simulink library "halout"  (R2021b)
settings: Solver=VariableStepAuto  StartTime=0.0  StopTime=10.0  RelTol=1e-3
undefined symbols (not defined in the file): C_TASK_5MS_S, FALSE, KHAL_CAN1FD1APS3E2E_flg, KHAL_CAN1FD1APS3TxReq_flg, KHAL_CAN1FD1VCU2E2E_flg, KHAL_CAN1FD1VCU2TxReq_flg, KHAL_CAN1FD1VCU3E2E_flg, KHAL_CAN1FD1VCU3TxReq_flg, KHAL_CAN1TxReq_flg, KHAL_CAN1VMCFCM1E2E_flg, KHAL_CAN1VMCFCM1TxReq_flg, KHAL_CAN2TxReq_flg, KHAL_CAN3FD3VCU1toNIDECTxReq_flg, KHAL_CAN3FD3VCU1TxReq_flg, KHAL_CAN3FD3VCU2E2E_flg, KHAL_CAN3FD3VCU2toNIDECE2E_flg, KHAL_CAN3FD3VCU2toNIDECTxReq_flg, KHAL_CAN3FD3VCU2TxReq_flg, KHAL_CAN3TxReq_flg, KHAL_CAN4FD4CE1000E2E_flg, KHAL_CAN4FD4CE1000TxReq_flg, KHAL_CAN4TxReq_flg, KHAL_CAN5TxReq_flg, KHAL_CAN6FD6APS3E2E_flg, KHAL_CAN6FD6APS3TxReq_flg, KHAL_CAN6FD6VCU2E2E_flg, KHAL_CAN6FD6VCU2TxReq_flg, KHAL_CAN6TxReq_flg, ONE_INT, TRUE, ZERO_INT
libraries: FVT_lib x551, simulink x244
(part 17 of 26)

== system halout/HAL_OUT/CAN2/FD2_C20_0_0x210/PASDRCR ==
  PASDRCR : Inport
  Data Type Conversion : DataTypeConversion  OutDataTypeStr=uint8  RndMeth=Round
  CAN2_PAS_D_RCR : Outport
  wires:
  Data Type Conversion/1 -> CAN2_PAS_D_RCR/1
  PASDRCR/1 -> Data Type Conversion/1

== system halout/HAL_OUT/CAN2/FD2_C20_0_0x210/PASDRML ==
  PASDRML : Inport
  Data Type Conversion : DataTypeConversion  OutDataTypeStr=uint8  RndMeth=Round
  CAN2_PAS_D_RML : Outport
  wires:
  Data Type Conversion/1 -> CAN2_PAS_D_RML/1
  PASDRML/1 -> Data Type Conversion/1

== system halout/HAL_OUT/CAN2/FD2_C20_0_0x210/PASDRMR ==
  PASDRMR : Inport
  Data Type Conversion : DataTypeConversion  OutDataTypeStr=uint8  RndMeth=Round
  CAN2_PAS_D_RMR : Outport
  wires:
  Data Type Conversion/1 -> CAN2_PAS_D_RMR/1
  PASDRMR/1 -> Data Type Conversion/1

== system halout/HAL_OUT/CAN2/FD2_C20_0_0x210/PASSNSRLayout ==
  PASSNSRLayout : Inport
  Data Type Conversion : DataTypeConversion  OutDataTypeStr=uint8  RndMeth=Round
  CAN2_PAS_SNSR_Layout : Outport
  wires:
  Data Type Conversion/1 -> CAN2_PAS_SNSR_Layout/1
  PASSNSRLayout/1 -> Data Type Conversion/1

== system halout/HAL_OUT/CAN2/FD2_C20_0_0x210/USSStaFCL ==
  USSStaFCL : Inport
  Data Type Conversion : DataTypeConversion  OutDataTypeStr=uint8  RndMeth=Round
  CAN2_USS_Sta_FCL : Outport
  wires:
  Data Type Conversion/1 -> CAN2_USS_Sta_FCL/1
  USSStaFCL/1 -> Data Type Conversion/1

== system halout/HAL_OUT/CAN2/FD2_C20_0_0x210/USSStaFCR ==
  USSStaFCR : Inport
  Data Type Conversion : DataTypeConversion  OutDataTypeStr=uint8  RndMeth=Round
  CAN2_USS_Sta_FCR : Outport
  wires:
  Data Type Conversion/1 -> CAN2_USS_Sta_FCR/1
  USSStaFCR/1 -> Data Type Conversion/1

== system halout/HAL_OUT/CAN2/FD2_C20_0_0x210/USSStaFLL ==
  USSStaFLL : Inport
  Data Type Conversion : DataTypeConversion  OutDataTypeStr=uint8  RndMeth=Round
  CAN2_USS_Sta_FLL : Outport
  wires:
  Data Type Conversion/1 -> CAN2_USS_Sta_FLL/1
  USSStaFLL/1 -> Data Type Conversion/1

== system halout/HAL_OUT/CAN2/FD2_C20_0_0x210/USSStaFLR ==
  USSStaFLR : Inport
  Data Type Conversion : DataTypeConversion  OutDataTypeStr=uint8  RndMeth=Round
  CAN2_USS_Sta_FLR : Outport
  wires:
  Data Type Conversion/1 -> CAN2_USS_Sta_FLR/1
  USSStaFLR/1 -> Data Type Conversion/1

== system halout/HAL_OUT/CAN2/FD2_C20_0_0x210/USSStaFML ==
  USSStaFML : Inport
  Data Type Conversion : DataTypeConversion  OutDataTypeStr=uint8  RndMeth=Round
  CAN2_USS_Sta_FML : Outport
  wires:
  Data Type Conversion/1 -> CAN2_USS_Sta_FML/1
  USSStaFML/1 -> Data Type Conversion/1

== system halout/HAL_OUT/CAN2/FD2_C20_0_0x210/USSStaFMR ==
  USSStaFMR : Inport
  Data Type Conversion : DataTypeConversion  OutDataTypeStr=uint8  RndMeth=Round
  CAN2_USS_Sta_FMR : Outport
  wires:
  Data Type Conversion/1 -> CAN2_USS_Sta_FMR/1
  USSStaFMR/1 -> Data Type Conversion/1

== system halout/HAL_OUT/CAN2/FD2_C20_0_0x210/USSStaRCL ==
  USSStaRCL : Inport
  Data Type Conversion : DataTypeConversion  OutDataTypeStr=uint8  RndMeth=Round
  CAN2_USS_Sta_RCL : Outport
  wires:
  Data Type Conversion/1 -> CAN2_USS_Sta_RCL/1
  USSStaRCL/1 -> Data Type Conversion/1

== system halout/HAL_OUT/CAN2/FD2_C20_0_0x210/USSStaRCR ==
  USSStaRCR : Inport
  Data Type Conversion : DataTypeConversion  OutDataTypeStr=uint8  RndMeth=Round
  CAN2_USS_Sta_RCR : Outport
  wires:
  Data Type Conversion/1 -> CAN2_USS_Sta_RCR/1
  USSStaRCR/1 -> Data Type Conversion/1

== system halout/HAL_OUT/CAN2/FD2_C20_0_0x210/USSStaRLL ==
  USSStaRLL : Inport
  Data Type Conversion : DataTypeConversion  OutDataTypeStr=uint8  RndMeth=Round
  CAN2_USS_Sta_RLL : Outport
  wires:
  Data Type Conversion/1 -> CAN2_USS_Sta_RLL/1
  USSStaRLL/1 -> Data Type Conversion/1

== system halout/HAL_OUT/CAN2/FD2_C20_0_0x210/USSStaRLR ==
  USSStaRLR : Inport
  Data Type Conversion : DataTypeConversion  OutDataTypeStr=uint8  RndMeth=Round
  CAN2_USS_Sta_RLR : Outport
  wires:
  Data Type Conversion/1 -> CAN2_USS_Sta_RLR/1
  USSStaRLR/1 -> Data Type Conversion/1

== system halout/HAL_OUT/CAN2/FD2_C20_0_0x210/USSStaRML ==
  USSStaRML : Inport
  Data Type Conversion : DataTypeConversion  OutDataTypeStr=uint8  RndMeth=Round
  CAN2_USS_Sta_RML : Outport
  wires:
  Data Type Conversion/1 -> CAN2_USS_Sta_RML/1
  USSStaRML/1 -> Data Type Conversion/1

== system halout/HAL_OUT/CAN2/FD2_C20_0_0x210/USSStaRMR ==
  USSStaRMR : Inport
  Data Type Conversion : DataTypeConversion  OutDataTypeStr=uint8  RndMeth=Round
  CAN2_USS_Sta_RMR : Outport
  wires:
  Data Type Conversion/1 -> CAN2_USS_Sta_RMR/1
  USSStaRMR/1 -> Data Type Conversion/1

== system halout/HAL_OUT/CAN2/FD2_C20_0_0x210/VMCVCUCCCrlSta ==
  VMCVCUCCCrlSta : Inport
  Data Type Conversion : DataTypeConversion  OutDataTypeStr=uint8  RndMeth=Round
  CAN2_VMC_VCU_CC_Crl_Sta : Outport
  wires:
  Data Type Conversion/1 -> CAN2_VMC_VCU_CC_Crl_Sta/1
  VMCVCUCCCrlSta/1 -> Data Type Conversion/1

== system halout/HAL_OUT/CAN2/FD2_C20_0_0x210/VMCVCUMSACrlSta ==
  VMCVCUMSACrlSta : Inport
  Data Type Conversion : DataTypeConversion  OutDataTypeStr=uint8  RndMeth=Round
  CAN2_VMC_VCU_MSA_Crl_Sta : Outport
  wires:
  Data Type Conversion/1 -> CAN2_VMC_VCU_MSA_Crl_Sta/1
  VMCVCUMSACrlSta/1 -> Data Type Conversion/1

== system halout/HAL_OUT/CAN2/FD2_CE100_0_0x117/APMDoorControlSta ==
  APMDoorControlSta : Inport
  Data Type Conversion : DataTypeConversion  OutDataTypeStr=uint8  RndMeth=Round
  CAN2_APMDoorControlSta : Outport
  wires:
  Data Type Conversion/1 -> CAN2_APMDoorControlSta/1
  APMDoorControlSta/1 -> Data Type Conversion/1

== system halout/HAL_OUT/CAN2/FD2_CE100_0_0x117/ActAPSPosn ==
  ActAPSPosn : Inport
  Data Type Conversion : DataTypeConversion  OutDataTypeStr=uint8  RndMeth=Round
  convert_out : FVT_lib/hal/convert_out  gain=0.394  offset=0
  CAN2_ActAPSPosn : Outport
  wires:
  Data Type Conversion/1 -> CAN2_ActAPSPosn/1
  convert_out/1 -> Data Type Conversion/1
  ActAPSPosn/1 -> convert_out/1

== system halout/HAL_OUT/CAN2/FD2_CE100_0_0x117/AllDoorSW ==
  AllDoorSW : Inport
  Data Type Conversion : DataTypeConversion  OutDataTypeStr=uint8  RndMeth=Round
  CAN2_AllDoorSW : Outport
  wires:
  Data Type Conversion/1 -> CAN2_AllDoorSW/1
  AllDoorSW/1 -> Data Type Conversion/1

== system halout/HAL_OUT/CAN2/FD2_CE100_0_0x117/AntitheftSta ==
  AntitheftSta : Inport
  Data Type Conversion : DataTypeConversion  OutDataTypeStr=uint8  RndMeth=Round
  CAN2_AntitheftSta : Outport
  wires:
  Data Type Conversion/1 -> CAN2_AntitheftSta/1
  AntitheftSta/1 -> Data Type Conversion/1

== system halout/HAL_OUT/CAN2/FD2_CE100_0_0x117/BCMDoorLockSta ==
  BCMDoorLockSta : Inport
  Data Type Conversion : DataTypeConversion  OutDataTypeStr=uint8  RndMeth=Round
  CAN2_BCM_DoorLock_Sta : Outport
  wires:
  Data Type Conversion/1 -> CAN2_BCM_DoorLock_Sta/1
  BCMDoorLockSta/1 -> Data Type Conversion/1

== system halout/HAL_OUT/CAN2/FD2_CE100_0_0x117/BrakeLamp ==
  BrakeLamp : Inport
  Data Type Conversion : DataTypeConversion  OutDataTypeStr=uint8  RndMeth=Round
  CAN2_BrakeLamp : Outport
  wires:
  Data Type Conversion/1 -> CAN2_BrakeLamp/1
  BrakeLamp/1 -> Data Type Conversion/1

== system halout/HAL_OUT/CAN2/FD2_CE100_0_0x117/CCCrlSta ==
  CCCrlSta : Inport
  Data Type Conversion : DataTypeConversion  OutDataTypeStr=uint8  RndMeth=Round
  CAN2_CC_Crl_Sta : Outport
  wires:
  Data Type Conversion/1 -> CAN2_CC_Crl_Sta/1
  CCCrlSta/1 -> Data Type Conversion/1

== system halout/HAL_OUT/CAN2/FD2_CE100_0_0x117/CCMSASpdWar ==
  CCMSASpdWar : Inport
  Data Type Conversion : DataTypeConversion  OutDataTypeStr=uint8  RndMeth=Round
  CAN2_CCMSA_SpdWar : Outport
  wires:
  Data Type Conversion/1 -> CAN2_CCMSA_SpdWar/1
  CCMSASpdWar/1 -> Data Type Conversion/1

== system halout/HAL_OUT/CAN2/FD2_CE100_0_0x117/CCUACLampSts ==
  CCUACLampSts : Inport
  Data Type Conversion : DataTypeConversion  OutDataTypeStr=uint8  RndMeth=Round
  CAN2_CCU_ACLampSts : Outport
  wires:
  Data Type Conversion/1 -> CAN2_CCU_ACLampSts/1
  CCUACLampSts/1 -> Data Type Conversion/1

== system halout/HAL_OUT/CAN2/FD2_CE100_0_0x117/CCUACMaxLampSts ==
  CCUACMaxLampSts : Inport
  Data Type Conversion : DataTypeConversion  OutDataTypeStr=uint8  RndMeth=Round
  CAN2_CCU_ACMaxLampSts : Outport
  wires:
  Data Type Conversion/1 -> CAN2_CCU_ACMaxLampSts/1
  CCUACMaxLampSts/1 -> Data Type Conversion/1

== system halout/HAL_OUT/CAN2/FD2_CE100_0_0x117/CCUAutoLampSts ==
  CCUAutoLampSts : Inport
  Data Type Conversion : DataTypeConversion  OutDataTypeStr=uint8  RndMeth=Round
  CAN2_CCU_AutoLampSts : Outport
  wires:
  Data Type Conversion/1 -> CAN2_CCU_AutoLampSts/1
  CCUAutoLampSts/1 -> Data Type Conversion/1

== system halout/HAL_OUT/CAN2/FD2_CE100_0_0x117/CCUAutoMidLampSts ==
  CCUAutoMidLampSts : Inport
  Data Type Conversion : DataTypeConversion  OutDataTypeStr=uint8  RndMeth=Round
  CAN2_CCU_AutoMidLampSts : Outport
  wires:
  Data Type Conversion/1 -> CAN2_CCU_AutoMidLampSts/1
  CCUAutoMidLampSts/1 -> Data Type Conversion/1

== system halout/HAL_OUT/CAN2/FD2_CE100_0_0x117/CCUDispalyRequest ==
  CCUDispalyRequest : Inport
  Data Type Conversion : DataTypeConversion  OutDataTypeStr=uint8  RndMeth=Round
  CAN2_CCU_Dispaly_Request : Outport
  wires:
  Data Type Conversion/1 -> CAN2_CCU_Dispaly_Request/1
  CCUDispalyRequest/1 -> Data Type Conversion/1

== system halout/HAL_OUT/CAN2/FD2_CE100_0_0x117/CCUEcoSts ==
  CCUEcoSts : Inport
  Data Type Conversion : DataTypeConversion  OutDataTypeStr=uint8  RndMeth=Round
  CAN2_CCU_EcoSts : Outport
  wires:
  Data Type Conversion/1 -> CAN2_CCU_EcoSts/1
  CCUEcoSts/1 -> Data Type Conversion/1

== system halout/HAL_OUT/CAN2/FD2_CE100_0_0x117/CCUFrtOnOffLampSts ==
  CCUFrtOnOffLampSts : Inport
  Data Type Conversion : DataTypeConversion  OutDataTypeStr=uint8  RndMeth=Round
  CAN2_CCU_FrtOnOffLampSts : Outport
  wires:
  Data Type Conversion/1 -> CAN2_CCU_FrtOnOffLampSts/1
  CCUFrtOnOffLampSts/1 -> Data Type Conversion/1

== system halout/HAL_OUT/CAN2/FD2_CE100_0_0x117/CCURrOnOffLampSts ==
  CCURrOnOffLampSts : Inport
  Data Type Conversion : DataTypeConversion  OutDataTypeStr=uint8  RndMeth=Round
  CAN2_CCU_RrOnOffLampSts : Outport
  wires:
  Data Type Conversion/1 -> CAN2_CCU_RrOnOffLampSts/1
  CCURrOnOffLampSts/1 -> Data Type Conversion/1

== system halout/HAL_OUT/CAN2/FD2_CE100_0_0x117/CCUSyncLampSts ==
  CCUSyncLampSts : Inport
  Data Type Conversion : DataTypeConversion  OutDataTypeStr=uint8  RndMeth=Round
  CAN2_CCU_SyncLampSts : Outport
  wires:
  Data Type Conversion/1 -> CAN2_CCU_SyncLampSts/1
  CCUSyncLampSts/1 -> Data Type Conversion/1

== system halout/HAL_OUT/CAN2/FD2_CE100_0_0x117/CoastDwModeStaChk ==
  CoastDwModeStaChk : Inport
  Data Type Conversion : DataTypeConversion  OutDataTypeStr=uint8  RndMeth=Round
  CAN2_CoastDwModeStaChk : Outport
  wires:
  Data Type Conversion/1 -> CAN2_CoastDwModeStaChk/1
  CoastDwModeStaChk/1 -> Data Type Conversion/1

== system halout/HAL_OUT/CAN2/FD2_CE100_0_0x117/CreepSWSta ==
  CreepSWSta : Inport
  Data Type Conversion : DataTypeConversion  OutDataTypeStr=uint8  RndMeth=Round
  CAN2_CreepSW_Sta : Outport
  wires:
  Data Type Conversion/1 -> CAN2_CreepSW_Sta/1
  CreepSWSta/1 -> Data Type Conversion/1

== system halout/HAL_OUT/CAN2/FD2_CE100_0_0x117/DISCButtSta ==
  DISCButtSta : Inport
  Data Type Conversion : DataTypeConversion  OutDataTypeStr=uint8  RndMeth=Round
  CAN2_DISC_ButtSta : Outport
  wires:
  Data Type Conversion/1 -> CAN2_DISC_ButtSta/1
  DISCButtSta/1 -> Data Type Conversion/1

== system halout/HAL_OUT/CAN2/FD2_CE100_0_0x117/DISCSta ==
  DISCSta : Inport
  Data Type Conversion : DataTypeConversion  OutDataTypeStr=uint8  RndMeth=Round
  CAN2_DISC_Sta : Outport
  wires:
  Data Type Conversion/1 -> CAN2_DISC_Sta/1
  DISCSta/1 -> Data Type Conversion/1

== system halout/HAL_OUT/CAN2/FD2_CE100_0_0x117/DemoModeStaChk ==
  DemoModeStaChk : Inport
  Data Type Conversion : DataTypeConversion  OutDataTypeStr=uint8  RndMeth=Round
  CAN2_DemoModeStaChk : Outport
  wires:
  Data Type Conversion/1 -> CAN2_DemoModeStaChk/1
  DemoModeStaChk/1 -> Data Type Conversion/1

== system halout/HAL_OUT/CAN2/FD2_CE100_0_0x117/Dimmer ==
  Dimmer : Inport
  Data Type Conversion : DataTypeConversion  OutDataTypeStr=uint8  RndMeth=Round
  CAN2_Dimmer : Outport
  wires:
  Data Type Conversion/1 -> CAN2_Dimmer/1
  Dimmer/1 -> Data Type Conversion/1

== system halout/HAL_OUT/CAN2/FD2_CE100_0_0x117/DimmerEN ==
  DimmerEN : Inport
  Data Type Conversion : DataTypeConversion  OutDataTypeStr=uint8  RndMeth=Round
  CAN2_DimmerEN : Outport
  wires:
  Data Type Conversion/1 -> CAN2_DimmerEN/1
  DimmerEN/1 -> Data Type Conversion/1

== system halout/HAL_OUT/CAN2/FD2_CE100_0_0x117/DisengagePFail ==
  DisengagePFail : Inport
  Data Type Conversion : DataTypeConversion  OutDataTypeStr=uint8  RndMeth=Round
  CAN2_DisengageP_Fail : Outport
  wires:
  Data Type Conversion/1 -> CAN2_DisengageP_Fail/1
  DisengagePFail/1 -> Data Type Conversion/1

== system halout/HAL_OUT/CAN2/FD2_CE100_0_0x117/DoorLockIND ==
  DoorLockIND : Inport
  Data Type Conversion : DataTypeConversion  OutDataTypeStr=uint8  RndMeth=Round
  CAN2_DoorLockIND : Outport
  wires:
  Data Type Conversion/1 -> CAN2_DoorLockIND/1
  DoorLockIND/1 -> Data Type Conversion/1

== system halout/HAL_OUT/CAN2/FD2_CE100_0_0x117/DrDoorSW ==
  DrDoorSW : Inport
  Data Type Conversion : DataTypeConversion  OutDataTypeStr=uint8  RndMeth=Round
  CAN2_DrDoorSW : Outport
  wires:
  Data Type Conversion/1 -> CAN2_DrDoorSW/1
  DrDoorSW/1 -> Data Type Conversion/1

== system halout/HAL_OUT/CAN2/FD2_CE100_0_0x117/DrSeatSta ==
  DrSeatSta : Inport
  Data Type Conversion : DataTypeConversion  OutDataTypeStr=uint8  RndMeth=Round
  CAN2_Dr_SeatSta : Outport
  wires:
  Data Type Conversion/1 -> CAN2_Dr_SeatSta/1
  DrSeatSta/1 -> Data Type Conversion/1

== system halout/HAL_OUT/CAN2/FD2_CE100_0_0x117/DynoModeStaChk ==
  DynoModeStaChk : Inport
  Data Type Conversion : DataTypeConversion  OutDataTypeStr=uint8  RndMeth=Round
  CAN2_DynoModeStaChk : Outport
  wires:
  Data Type Conversion/1 -> CAN2_DynoModeStaChk/1
  DynoModeStaChk/1 -> Data Type Conversion/1

== system halout/HAL_OUT/CAN2/FD2_CE100_0_0x117/EDriveSysErrAccPedalErr ==
  EDriveSysErrAccPedalErr : Inport
  Data Type Conversion : DataTypeConversion  OutDataTypeStr=uint8  RndMeth=Round
  CAN2_EDriveSysErr_AccPedalErr : Outport
  wires:
  Data Type Conversion/1 -> CAN2_EDriveSysErr_AccPedalErr/1
  EDriveSysErrAccPedalErr/1 -> Data Type Conversion/1

== system halout/HAL_OUT/CAN2/FD2_CE100_0_0x117/EDriveSysErrMCUErr ==
  EDriveSysErrMCUErr : Inport
  Data Type Conversion : DataTypeConversion  OutDataTypeStr=uint8  RndMeth=Round
  CAN2_EDriveSysErr_MCUErr : Outport
  wires:
  Data Type Conversion/1 -> CAN2_EDriveSysErr_MCUErr/1
  EDriveSysErrMCUErr/1 -> Data Type Conversion/1

== system halout/HAL_OUT/CAN2/FD2_CE100_0_0x117/EDriveSysErrShifterErr ==
  EDriveSysErrShifterErr : Inport
  Data Type Conversion : DataTypeConversion  OutDataTypeStr=uint8  RndMeth=Round
  CAN2_EDriveSysErr_ShifterErr : Outport
  wires:
  Data Type Conversion/1 -> CAN2_EDriveSysErr_ShifterErr/1
  EDriveSysErrShifterErr/1 -> Data Type Conversion/1

== system halout/HAL_OUT/CAN2/FD2_CE100_0_0x117/EDriveSysErrVCUErr ==
  EDriveSysErrVCUErr : Inport
  Data Type Conversion : DataTypeConversion  OutDataTypeStr=uint8  RndMeth=Round
  CAN2_EDriveSysErr_VCUErr : Outport
  wires:
  Data Type Conversion/1 -> CAN2_EDriveSysErr_VCUErr/1
  EDriveSysErrVCUErr/1 -> Data Type Conversion/1

== system halout/HAL_OUT/CAN2/FD2_CE100_0_0x117/EVDriveMode ==
  EVDriveMode : Inport
  Data Type Conversion : DataTypeConversion  OutDataTypeStr=uint8  RndMeth=Round
  CAN2_EVDriveMode : Outport
  wires:
  Data Type Conversion/1 -> CAN2_EVDriveMode/1
  EVDriveMode/1 -> Data Type Conversion/1

== system halout/HAL_OUT/CAN2/FD2_CE100_0_0x117/EngAGSCloseSta ==
  EngAGSCloseSta : Inport
  Data Type Conversion : DataTypeConversion  OutDataTypeStr=uint8  RndMeth=Round
  CAN2_Eng_AGSCloseSta : Outport
  wires:
  Data Type Conversion/1 -> CAN2_Eng_AGSCloseSta/1
  EngAGSCloseSta/1 -> Data Type Conversion/1

== system halout/HAL_OUT/CAN2/FD2_CE100_0_0x117/EngActvDmpDisabSta ==
  EngActvDmpDisabSta : Inport
  Data Type Conversion : DataTypeConversion  OutDataTypeStr=uint8  RndMeth=Round
  CAN2_Eng_ActvDmpDisabSta : Outport
  wires:
  Data Type Conversion/1 -> CAN2_Eng_ActvDmpDisabSta/1
  EngActvDmpDisabSta/1 -> Data Type Conversion/1

== system halout/HAL_OUT/CAN2/FD2_CE100_0_0x117/EngCoastDwSta ==
  EngCoastDwSta : Inport
  Data Type Conversion : DataTypeConversion  OutDataTypeStr=uint8  RndMeth=Round
  CAN2_Eng_CoastDwSta : Outport
  wires:
  Data Type Conversion/1 -> CAN2_Eng_CoastDwSta/1
  EngCoastDwSta/1 -> Data Type Conversion/1

== system halout/HAL_OUT/CAN2/FD2_CE100_0_0x117/EngPwrLockSta ==
  EngPwrLockSta : Inport
  Data Type Conversion : DataTypeConversion  OutDataTypeStr=uint8  RndMeth=Round
  CAN2_Eng_PwrLockSta : Outport
  wires:
  Data Type Conversion/1 -> CAN2_Eng_PwrLockSta/1
  EngPwrLockSta/1 -> Data Type Conversion/1

== system halout/HAL_OUT/CAN2/FD2_CE100_0_0x117/EngagePFail ==
  EngagePFail : Inport
  Data Type Conversion : DataTypeConversion  OutDataTypeStr=uint8  RndMeth=Round
  CAN2_EngageP_Fail : Outport
  wires:
  Data Type Conversion/1 -> CAN2_EngageP_Fail/1
  EngagePFail/1 -> Data Type Conversion/1

== system halout/HAL_OUT/CAN2/FD2_CE100_0_0x117/FDABSWarning ==
  FDABSWarning : Inport
  Data Type Conversion : DataTypeConversion  OutDataTypeStr=uint8  RndMeth=Round
  CAN2_FD_ABS_Warning : Outport
  wires:
  Data Type Conversion/1 -> CAN2_FD_ABS_Warning/1
  FDABSWarning/1 -> Data Type Conversion/1

== system halout/HAL_OUT/CAN2/FD2_CE100_0_0x117/FDAGSCmd ==
  FDAGSCmd : Inport
  Data Type Conversion : DataTypeConversion  OutDataTypeStr=uint8  RndMeth=Round
  CAN2_FD_AGS_Cmd : Outport
  wires:
  Data Type Conversion/1 -> CAN2_FD_AGS_Cmd/1
  FDAGSCmd/1 -> Data Type Conversion/1

== system halout/HAL_OUT/CAN2/FD2_CE100_0_0x117/FDBatteryChargeWarning ==
  FDBatteryChargeWarning : Inport
  Data Type Conversion : DataTypeConversion  OutDataTypeStr=uint8  RndMeth=Round
  CAN2_FD_Battery_Charge_Warning : Outport
  wires:
  Data Type Conversion/1 -> CAN2_FD_Battery_Charge_Warning/1
  FDBatteryChargeWarning/1 -> Data Type Conversion/1

== system halout/HAL_OUT/CAN2/FD2_CE100_0_0x117/FDCBCMAutoWipHSpdENSta ==
  FDCBCMAutoWipHSpdENSta : Inport
  Data Type Conversion : DataTypeConversion  OutDataTypeStr=uint8  RndMeth=Round
  CAN2_FDC_BCM_AutoWipHSpdEN_Sta : Outport
  wires:
  Data Type Conversion/1 -> CAN2_FDC_BCM_AutoWipHSpdEN_Sta/1
  FDCBCMAutoWipHSpdENSta/1 -> Data Type Conversion/1

== system halout/HAL_OUT/CAN2/FD2_CE100_0_0x117/FDCBCMHMIKey1FuncSta ==
  FDCBCMHMIKey1FuncSta : Inport
  Data Type Conversion : DataTypeConversion  OutDataTypeStr=uint8  RndMeth=Round
  CAN2_FDC_BCM_HMIKey1Func_Sta : Outport
  wires:
  Data Type Conversion/1 -> CAN2_FDC_BCM_HMIKey1Func_Sta/1
  FDCBCMHMIKey1FuncSta/1 -> Data Type Conversion/1

== system halout/HAL_OUT/CAN2/FD2_CE100_0_0x117/FDCBCMHMIKey2FuncSta ==
  FDCBCMHMIKey2FuncSta : Inport
  Data Type Conversion : DataTypeConversion  OutDataTypeStr=uint8  RndMeth=Round
  CAN2_FDC_BCM_HMIKey2Func_Sta : Outport
  wires:
  Data Type Conversion/1 -> CAN2_FDC_BCM_HMIKey2Func_Sta/1
  FDCBCMHMIKey2FuncSta/1 -> Data Type Conversion/1

== system halout/HAL_OUT/CAN2/FD2_CE100_0_0x117/FDCBCMHMIKey3FuncSta ==
  FDCBCMHMIKey3FuncSta : Inport
  Data Type Conversion : DataTypeConversion  OutDataTypeStr=uint8  RndMeth=Round
  CAN2_FDC_BCM_HMIKey3Func_Sta : Outport
  wires:
  Data Type Conversion/1 -> CAN2_FDC_BCM_HMIKey3Func_Sta/1
  FDCBCMHMIKey3FuncSta/1 -> Data Type Conversion/1

== system halout/HAL_OUT/CAN2/FD2_CE100_0_0x117/FDCBCMHMIKey4FuncSta ==
  FDCBCMHMIKey4FuncSta : Inport
  Data Type Conversion : DataTypeConversion  OutDataTypeStr=uint8  RndMeth=Round
  CAN2_FDC_BCM_HMIKey4Func_Sta : Outport
  wires:
  Data Type Conversion/1 -> CAN2_FDC_BCM_HMIKey4Func_Sta/1
  FDCBCMHMIKey4FuncSta/1 -> Data Type Conversion/1

== system halout/HAL_OUT/CAN2/FD2_CE100_0_0x117/FDCBCMHMIKey5FuncSta ==
  FDCBCMHMIKey5FuncSta : Inport
  Data Type Conversion : DataTypeConversion  OutDataTypeStr=uint8  RndMeth=Round
  CAN2_FDC_BCM_HMIKey5Func_Sta : Outport
  wires:
  Data Type Conversion/1 -> CAN2_FDC_BCM_HMIKey5Func_Sta/1
  FDCBCMHMIKey5FuncSta/1 -> Data Type Conversion/1

== system halout/HAL_OUT/CAN2/FD2_CE100_0_0x117/FDCBCMHMIKey6FuncSta ==
  FDCBCMHMIKey6FuncSta : Inport
  Data Type Conversion : DataTypeConversion  OutDataTypeStr=uint8  RndMeth=Round
  CAN2_FDC_BCM_HMIKey6Func_Sta : Outport
  wires:
  Data Type Conversion/1 -> CAN2_FDC_BCM_HMIKey6Func_Sta/1
  FDCBCMHMIKey6FuncSta/1 -> Data Type Conversion/1

== system halout/HAL_OUT/CAN2/FD2_CE100_0_0x117/FDCBCMHMIKey7FuncSta ==
  FDCBCMHMIKey7FuncSta : Inport
  Data Type Conversion : DataTypeConversion  OutDataTypeStr=uint8  RndMeth=Round
  CAN2_FDC_BCM_HMIKey7Func_Sta : Outport
  wires:
  Data Type Conversion/1 -> CAN2_FDC_BCM_HMIKey7Func_Sta/1
  FDCBCMHMIKey7FuncSta/1 -> Data Type Conversion/1

== system halout/HAL_OUT/CAN2/FD2_CE100_0_0x117/FDCBCMHMIKey8FuncSta ==
  FDCBCMHMIKey8FuncSta : Inport
  Data Type Conversion : DataTypeConversion  OutDataTypeStr=uint8  RndMeth=Round
  CAN2_FDC_BCM_HMIKey8Func_Sta : Outport
  wires:
  Data Type Conversion/1 -> CAN2_FDC_BCM_HMIKey8Func_Sta/1
  FDCBCMHMIKey8FuncSta/1 -> Data Type Conversion/1

== system halout/HAL_OUT/CAN2/FD2_CE100_0_0x117/FDCRAPSErrWarnSta ==
  FDCRAPSErrWarnSta : Inport
  Data Type Conversion : DataTypeConversion  OutDataTypeStr=uint8  RndMeth=Round
  CAN2_FDC_RAPS_ErrWarn_Sta : Outport
  wires:
  Data Type Conversion/1 -> CAN2_FDC_RAPS_ErrWarn_Sta/1
  FDCRAPSErrWarnSta/1 -> Data Type Conversion/1

== system halout/HAL_OUT/CAN2/FD2_CE100_0_0x117/FDCTHCMCLEVentYSta ==
  FDCTHCMCLEVentYSta : Inport
  Data Type Conversion : DataTypeConversion  OutDataTypeStr=uint8  RndMeth=Round
  CAN2_FDC_THCM_CLEVentY_Sta : Outport
  wires:
  Data Type Conversion/1 -> CAN2_FDC_THCM_CLEVentY_Sta/1
  FDCTHCMCLEVentYSta/1 -> Data Type Conversion/1

== system halout/HAL_OUT/CAN2/FD2_CE100_0_0x117/FDCTHCMCLEVentZSta ==
  FDCTHCMCLEVentZSta : Inport
  Data Type Conversion : DataTypeConversion  OutDataTypeStr=uint8  RndMeth=Round
  CAN2_FDC_THCM_CLEVentZ_Sta : Outport
  wires:
  Data Type Conversion/1 -> CAN2_FDC_THCM_CLEVentZ_Sta/1
  FDCTHCMCLEVentZSta/1 -> Data Type Conversion/1

== system halout/HAL_OUT/CAN2/FD2_CE100_0_0x117/FDCTHCMCLVentSta ==
  FDCTHCMCLVentSta : Inport
  Data Type Conversion : DataTypeConversion  OutDataTypeStr=uint8  RndMeth=Round
  CAN2_FDC_THCM_CLVent_Sta : Outport
  wires:
  Data Type Conversion/1 -> CAN2_FDC_THCM_CLVent_Sta/1
  FDCTHCMCLVentSta/1 -> Data Type Conversion/1

== system halout/HAL_OUT/CAN2/FD2_CE100_0_0x117/FDCTHCMCREVentYSta ==
  FDCTHCMCREVentYSta : Inport
  Data Type Conversion : DataTypeConversion  OutDataTypeStr=uint8  RndMeth=Round
  CAN2_FDC_THCM_CREVentY_Sta : Outport
  wires:
  Data Type Conversion/1 -> CAN2_FDC_THCM_CREVentY_Sta/1
  FDCTHCMCREVentYSta/1 -> Data Type Conversion/1

== system halout/HAL_OUT/CAN2/FD2_CE100_0_0x117/FDCTHCMCREVentZSta ==
  FDCTHCMCREVentZSta : Inport
  Data Type Conversion : DataTypeConversion  OutDataTypeStr=uint8  RndMeth=Round
  CAN2_FDC_THCM_CREVentZ_Sta : Outport
  wires:
  Data Type Conversion/1 -> CAN2_FDC_THCM_CREVentZ_Sta/1
  FDCTHCMCREVentZSta/1 -> Data Type Conversion/1

== system halout/HAL_OUT/CAN2/FD2_CE100_0_0x117/FDCTHCMCRVentSta ==
  FDCTHCMCRVentSta : Inport
  Data Type Conversion : DataTypeConversion  OutDataTypeStr=uint8  RndMeth=Round
  CAN2_FDC_THCM_CRVent_Sta : Outport
  wires:
  Data Type Conversion/1 -> CAN2_FDC_THCM_CRVent_Sta/1
  FDCTHCMCRVentSta/1 -> Data Type Conversion/1

== system halout/HAL_OUT/CAN2/FD2_CE100_0_0x117/FDCTHCMLEVentModeSta ==
  FDCTHCMLEVentModeSta : Inport
  Data Type Conversion : DataTypeConversion  OutDataTypeStr=uint8  RndMeth=Round
  CAN2_FDC_THCM_LEVentMode_Sta : Outport
  wires:
  Data Type Conversion/1 -> CAN2_FDC_THCM_LEVentMode_Sta/1
  FDCTHCMLEVentModeSta/1 -> Data Type Conversion/1

== system halout/HAL_OUT/CAN2/FD2_CE100_0_0x117/FDCTHCMLEVentYSta ==
  FDCTHCMLEVentYSta : Inport
  Data Type Conversion : DataTypeConversion  OutDataTypeStr=uint8  RndMeth=Round
  CAN2_FDC_THCM_LEVentY_Sta : Outport
  wires:
  Data Type Conversion/1 -> CAN2_FDC_THCM_LEVentY_Sta/1
  FDCTHCMLEVentYSta/1 -> Data Type Conversion/1

== system halout/HAL_OUT/CAN2/FD2_CE100_0_0x117/FDCTHCMLEVentZSta ==
  FDCTHCMLEVentZSta : Inport
  Data Type Conversion : DataTypeConversion  OutDataTypeStr=uint8  RndMeth=Round
  CAN2_FDC_THCM_LEVentZ_Sta : Outport
  wires:
  Data Type Conversion/1 -> CAN2_FDC_THCM_LEVentZ_Sta/1
  FDCTHCMLEVentZSta/1 -> Data Type Conversion/1

== system halout/HAL_OUT/CAN2/FD2_CE100_0_0x117/FDCTHCMLVentSta ==
  FDCTHCMLVentSta : Inport
  Data Type Conversion : DataTypeConversion  OutDataTypeStr=uint8  RndMeth=Round
  CAN2_FDC_THCM_LVent_Sta : Outport
  wires:
  Data Type Conversion/1 -> CAN2_FDC_THCM_LVent_Sta/1
  FDCTHCMLVentSta/1 -> Data Type Conversion/1

== system halout/HAL_OUT/CAN2/FD2_CE100_0_0x117/FDCTHCMPreWPTCHeatSta ==
  FDCTHCMPreWPTCHeatSta : Inport
  Data Type Conversion : DataTypeConversion  OutDataTypeStr=uint8  RndMeth=Round
  CAN2_FDC_THCM_PreWPTCHeat_Sta : Outport
  wires:
  Data Type Conversion/1 -> CAN2_FDC_THCM_PreWPTCHeat_Sta/1
  FDCTHCMPreWPTCHeatSta/1 -> Data Type Conversion/1

== system halout/HAL_OUT/CAN2/FD2_CE100_0_0x117/FDCTHCMREVentModeSta ==
  FDCTHCMREVentModeSta : Inport
  Data Type Conversion : DataTypeConversion  OutDataTypeStr=uint8  RndMeth=Round
  CAN2_FDC_THCM_REVentMode_Sta : Outport
  wires:
  Data Type Conversion/1 -> CAN2_FDC_THCM_REVentMode_Sta/1
  FDCTHCMREVentModeSta/1 -> Data Type Conversion/1

== system halout/HAL_OUT/CAN2/FD2_CE100_0_0x117/FDCTHCMREVentYSta ==
  FDCTHCMREVentYSta : Inport
  Data Type Conversion : DataTypeConversion  OutDataTypeStr=uint8  RndMeth=Round
  CAN2_FDC_THCM_REVentY_Sta : Outport
  wires:
  Data Type Conversion/1 -> CAN2_FDC_THCM_REVentY_Sta/1
  FDCTHCMREVentYSta/1 -> Data Type Conversion/1

== system halout/HAL_OUT/CAN2/FD2_CE100_0_0x117/FDCTHCMREVentZSta ==
  FDCTHCMREVentZSta : Inport
  Data Type Conversion : DataTypeConversion  OutDataTypeStr=uint8  RndMeth=Round
  CAN2_FDC_THCM_REVentZ_Sta : Outport
  wires:
  Data Type Conversion/1 -> CAN2_FDC_THCM_REVentZ_Sta/1
  FDCTHCMREVentZSta/1 -> Data Type Conversion/1

== system halout/HAL_OUT/CAN2/FD2_CE100_0_0x117/FDCTHCMRVentSta ==
  FDCTHCMRVentSta : Inport
  Data Type Conversion : DataTypeConversion  OutDataTypeStr=uint8  RndMeth=Round
  CAN2_FDC_THCM_RVent_Sta : Outport
  wires:
  Data Type Conversion/1 -> CAN2_FDC_THCM_RVent_Sta/1
  FDCTHCMRVentSta/1 -> Data Type Conversion/1

== system halout/HAL_OUT/CAN2/FD2_CE100_0_0x117/FDCV2LIVIV2LDischargCmd ==
  FDCV2LIVIV2LDischargCmd : Inport
  Data Type Conversion : DataTypeConversion  OutDataTypeStr=uint8  RndMeth=Round
  CAN2_FDC_V2L_IVIV2LDischarg_Cmd : Outport
  wires:
  Data Type Conversion/1 -> CAN2_FDC_V2L_IVIV2LDischarg_Cmd/1
  FDCV2LIVIV2LDischargCmd/1 -> Data Type Conversion/1

== system halout/HAL_OUT/CAN2/FD2_CE100_0_0x117/FDCVCULVChrgFreqSta ==
  FDCVCULVChrgFreqSta : Inport
  Data Type Conversion : DataTypeConversion  OutDataTypeStr=uint8  RndMeth=Round
  CAN2_FDC_VCU_LVChrgFreq_Sta : Outport
  wires:
  Data Type Conversion/1 -> CAN2_FDC_VCU_LVChrgFreq_Sta/1
  FDCVCULVChrgFreqSta/1 -> Data Type Conversion/1

== system halout/HAL_OUT/CAN2/FD2_CE100_0_0x117/FDCVCULVStaDropQuickSta ==
  FDCVCULVStaDropQuickSta : Inport
  Data Type Conversion : DataTypeConversion  OutDataTypeStr=uint8  RndMeth=Round
  CAN2_FDC_VCU_LVStaDropQuick_Sta : Outport
  wires:
  Data Type Conversion/1 -> CAN2_FDC_VCU_LVStaDropQuick_Sta/1
  FDCVCULVStaDropQuickSta/1 -> Data Type Conversion/1

== system halout/HAL_OUT/CAN2/FD2_CE100_0_0x117/FDCVCULVStaTooLowSta ==
  FDCVCULVStaTooLowSta : Inport
  Data Type Conversion : DataTypeConversion  OutDataTypeStr=uint8  RndMeth=Round
  CAN2_FDC_VCU_LVStaTooLow_Sta : Outport
  wires:
  Data Type Conversion/1 -> CAN2_FDC_VCU_LVStaTooLow_Sta/1
  FDCVCULVStaTooLowSta/1 -> Data Type Conversion/1

== system halout/HAL_OUT/CAN2/FD2_CE100_0_0x117/FDCVCUPwrSaveReqCmd ==
  FDCVCUPwrSaveReqCmd : Inport
  Data Type Conversion : DataTypeConversion  OutDataTypeStr=uint8  RndMeth=Round
  CAN2_FDC_VCU_PwrSaveReq_Cmd : Outport
  wires:
  Data Type Conversion/1 -> CAN2_FDC_VCU_PwrSaveReq_Cmd/1
  FDCVCUPwrSaveReqCmd/1 -> Data Type Conversion/1

== system halout/HAL_OUT/CAN2/FD2_CE100_0_0x117/FDCVCUTrailerDisOPDSta ==
  FDCVCUTrailerDisOPDSta : Inport
  Data Type Conversion : DataTypeConversion  OutDataTypeStr=uint8  RndMeth=Round
  CAN2_FDC_VCU_TrailerDisOPD_Sta : Outport
  wires:
  Data Type Conversion/1 -> CAN2_FDC_VCU_TrailerDisOPD_Sta/1
  FDCVCUTrailerDisOPDSta/1 -> Data Type Conversion/1

== system halout/HAL_OUT/CAN2/FD2_CE100_0_0x117/FDEBMErrSta ==
  FDEBMErrSta : Inport
  Data Type Conversion : DataTypeConversion  OutDataTypeStr=uint8  RndMeth=Round
  CAN2_FD_EBMErrSta : Outport
  wires:
  Data Type Conversion/1 -> CAN2_FD_EBMErrSta/1
  FDEBMErrSta/1 -> Data Type Conversion/1

== system halout/HAL_OUT/CAN2/FD2_CE100_0_0x117/FDEDriveSystem ==
  FDEDriveSystem : Inport
  Data Type Conversion : DataTypeConversion  OutDataTypeStr=uint8  RndMeth=Round
  CAN2_FD_EDrive_System : Outport
  wires:
  Data Type Conversion/1 -> CAN2_FD_EDrive_System/1
  FDEDriveSystem/1 -> Data Type Conversion/1

== system halout/HAL_OUT/CAN2/FD2_CE100_0_0x117/FDEPBError ==
  FDEPBError : Inport
  Data Type Conversion : DataTypeConversion  OutDataTypeStr=uint8  RndMeth=Round
  CAN2_FD_EPB_Error : Outport
  wires:
  Data Type Conversion/1 -> CAN2_FD_EPB_Error/1
  FDEPBError/1 -> Data Type Conversion/1

== system halout/HAL_OUT/CAN2/FD2_CE100_0_0x117/FDHVBatteryFault ==
  FDHVBatteryFault : Inport
  Data Type Conversion : DataTypeConversion  OutDataTypeStr=uint8  RndMeth=Round
  CAN2_FD_HV_Battery_Fault : Outport
  wires:
  Data Type Conversion/1 -> CAN2_FD_HV_Battery_Fault/1
  FDHVBatteryFault/1 -> Data Type Conversion/1

== system halout/HAL_OUT/CAN2/FD2_CE100_0_0x117/FDParkBrakeWarning ==
  FDParkBrakeWarning : Inport
  Data Type Conversion : DataTypeConversion  OutDataTypeStr=uint8  RndMeth=Round
  CAN2_FD_Park_Brake_Warning : Outport
  wires:
  Data Type Conversion/1 -> CAN2_FD_Park_Brake_Warning/1
  FDParkBrakeWarning/1 -> Data Type Conversion/1

== system halout/HAL_OUT/CAN2/FD2_CE100_0_0x117/FDPowerlimitation ==
  FDPowerlimitation : Inport
  Data Type Conversion : DataTypeConversion  OutDataTypeStr=uint8  RndMeth=Round
  CAN2_FD_Power_limitation : Outport
  wires:
  Data Type Conversion/1 -> CAN2_FD_Power_limitation/1
  FDPowerlimitation/1 -> Data Type Conversion/1

== system halout/HAL_OUT/CAN2/FD2_CE100_0_0x117/FDSteeringWarning ==
  FDSteeringWarning : Inport
  Data Type Conversion : DataTypeConversion  OutDataTypeStr=uint8  RndMeth=Round
  CAN2_FD_Steering_Warning : Outport
  wires:
  Data Type Conversion/1 -> CAN2_FD_Steering_Warning/1
  FDSteeringWarning/1 -> Data Type Conversion/1

== system halout/HAL_OUT/CAN2/FD2_CE100_0_0x117/FDTCSIndicator ==
  FDTCSIndicator : Inport
  Data Type Conversion : DataTypeConversion  OutDataTypeStr=uint8  RndMeth=Round
  CAN2_FD_TCS_Indicator : Outport
  wires:
  Data Type Conversion/1 -> CAN2_FD_TCS_Indicator/1
  FDTCSIndicator/1 -> Data Type Conversion/1

== system halout/HAL_OUT/CAN2/FD2_CE100_0_0x117/FDTelltaleFail ==
  FDTelltaleFail : Inport
  Data Type Conversion : DataTypeConversion  OutDataTypeStr=uint8  RndMeth=Round
  CAN2_FD_Telltale_Fail : Outport
  wires:
  Data Type Conversion/1 -> CAN2_FD_Telltale_Fail/1
  FDTelltaleFail/1 -> Data Type Conversion/1

== system halout/HAL_OUT/CAN2/FD2_CE100_0_0x117/FalseNPreventSta ==
  FalseNPreventSta : Inport
  Data Type Conversion : DataTypeConversion  OutDataTypeStr=uint8  RndMeth=Round
  CAN2_FalseNPrevent_Sta : Outport
  wires:
  Data Type Conversion/1 -> CAN2_FalseNPrevent_Sta/1
  FalseNPreventSta/1 -> Data Type Conversion/1

== system halout/HAL_OUT/CAN2/FD2_CE100_0_0x117/FeatSetSpdFinalraw32 ==
  FeatSetSpdFinalraw32 : Inport
  Data Type Conversion : DataTypeConversion  OutDataTypeStr=uint8  RndMeth=Round
  CAN2_FeatSetSpdFinal_raw32 : Outport
  wires:
  Data Type Conversion/1 -> CAN2_FeatSetSpdFinal_raw32/1
  FeatSetSpdFinalraw32/1 -> Data Type Conversion/1

== system halout/HAL_OUT/CAN2/FD2_CE100_0_0x117/FollowMe ==
  FollowMe : Inport
  Data Type Conversion : DataTypeConversion  OutDataTypeStr=uint8  RndMeth=Round
  CAN2_FollowMe : Outport
  wires:
  Data Type Conversion/1 -> CAN2_FollowMe/1
  FollowMe/1 -> Data Type Conversion/1

== system halout/HAL_OUT/CAN2/FD2_CE100_0_0x117/FrFogLamp ==
  FrFogLamp : Inport
  Data Type Conversion : DataTypeConversion  OutDataTypeStr=uint8  RndMeth=Round
  CAN2_Fr_FogLamp : Outport
  wires:
  Data Type Conversion/1 -> CAN2_Fr_FogLamp/1
  FrFogLamp/1 -> Data Type Conversion/1

== system halout/HAL_OUT/CAN2/FD2_CE100_0_0x117/HBeam ==
  HBeam : Inport
  Data Type Conversion : DataTypeConversion  OutDataTypeStr=uint8  RndMeth=Round
  CAN2_H_Beam : Outport
  wires:
  Data Type Conversion/1 -> CAN2_H_Beam/1
  HBeam/1 -> Data Type Conversion/1

== system halout/HAL_OUT/CAN2/FD2_CE100_0_0x117/HVRlyOpFail ==
  HVRlyOpFail : Inport
  Data Type Conversion : DataTypeConversion  OutDataTypeStr=uint8  RndMeth=Round
  CAN2_HVRlyOpFail : Outport
  wires:
  Data Type Conversion/1 -> CAN2_HVRlyOpFail/1
  HVRlyOpFail/1 -> Data Type Conversion/1

== system halout/HAL_OUT/CAN2/FD2_CE100_0_0x117/HVSysErrIsolationErr ==
  HVSysErrIsolationErr : Inport
  Data Type Conversion : DataTypeConversion  OutDataTypeStr=uint8  RndMeth=Round
  CAN2_HVSysErr_IsolationErr : Outport
  wires:
  Data Type Conversion/1 -> CAN2_HVSysErr_IsolationErr/1
  HVSysErrIsolationErr/1 -> Data Type Conversion/1

== system halout/HAL_OUT/CAN2/FD2_CE100_0_0x117/HVSysErrPackErr ==
  HVSysErrPackErr : Inport
  Data Type Conversion : DataTypeConversion  OutDataTypeStr=uint8  RndMeth=Round
  CAN2_HVSysErr_PackErr : Outport
  wires:
  Data Type Conversion/1 -> CAN2_HVSysErr_PackErr/1
  HVSysErrPackErr/1 -> Data Type Conversion/1

== system halout/HAL_OUT/CAN2/FD2_CE100_0_0x117/HVSysErrRelayErr ==
  HVSysErrRelayErr : Inport
  Data Type Conversion : DataTypeConversion  OutDataTypeStr=uint8  RndMeth=Round
  CAN2_HVSysErr_RelayErr : Outport
  wires:
  Data Type Conversion/1 -> CAN2_HVSysErr_RelayErr/1
  HVSysErrRelayErr/1 -> Data Type Conversion/1

== system halout/HAL_OUT/CAN2/FD2_CE100_0_0x117/HazardSW ==
  HazardSW : Inport
  Data Type Conversion : DataTypeConversion  OutDataTypeStr=uint8  RndMeth=Round
  CAN2_HazardSW : Outport
  wires:
  Data Type Conversion/1 -> CAN2_HazardSW/1
  HazardSW/1 -> Data Type Conversion/1

== system halout/HAL_OUT/CAN2/FD2_CE100_0_0x117/HoodSW ==
  HoodSW : Inport
  Data Type Conversion : DataTypeConversion  OutDataTypeStr=uint8  RndMeth=Round
  CAN2_HoodSW : Outport
  wires:
  Data Type Conversion/1 -> CAN2_HoodSW/1
  HoodSW/1 -> Data Type Conversion/1

== system halout/HAL_OUT/CAN2/FD2_CE100_0_0x117/LBSD ==
  LBSD : Inport
  Data Type Conversion : DataTypeConversion  OutDataTypeStr=uint8  RndMeth=Round
  CAN2_LBSD : Outport
  wires:
  Data Type Conversion/1 -> CAN2_LBSD/1
  LBSD/1 -> Data Type Conversion/1

== system halout/HAL_OUT/CAN2/FD2_CE100_0_0x117/LBeam ==
  LBeam : Inport
  Data Type Conversion : DataTypeConversion  OutDataTypeStr=uint8  RndMeth=Round
  CAN2_L_Beam : Outport
  wires:
  Data Type Conversion/1 -> CAN2_L_Beam/1
  LBeam/1 -> Data Type Conversion/1

== system halout/HAL_OUT/CAN2/FD2_CE100_0_0x117/LDRL ==
  LDRL : Inport
  Data Type Conversion : DataTypeConversion  OutDataTypeStr=uint8  RndMeth=Round
  CAN2_LDRL : Outport
  wires:
  Data Type Conversion/1 -> CAN2_LDRL/1
  LDRL/1 -> Data Type Conversion/1

== system halout/HAL_OUT/CAN2/FD2_CE100_0_0x117/LTurnLP ==
  LTurnLP : Inport
  Data Type Conversion : DataTypeConversion  OutDataTypeStr=uint8  RndMeth=Round
  CAN2_LTurnLP : Outport
  wires:
  Data Type Conversion/1 -> CAN2_LTurnLP/1
  LTurnLP/1 -> Data Type Conversion/1

== system halout/HAL_OUT/CAN2/FD2_CE100_0_0x117/LVChrgFuncStaChk ==
  LVChrgFuncStaChk : Inport
  Data Type Conversion : DataTypeConversion  OutDataTypeStr=uint8  RndMeth=Round
  CAN2_LVChrgFuncStaChk : Outport
  wires:
  Data Type Conversion/1 -> CAN2_LVChrgFuncStaChk/1
  LVChrgFuncStaChk/1 -> Data Type Conversion/1

== system halout/HAL_OUT/CAN2/FD2_CE100_0_0x117/LVSilentChrgReq ==
  LVSilentChrgReq : Inport
  Data Type Conversion : DataTypeConversion  OutDataTypeStr=uint8  RndMeth=Round
  CAN2_LVSilentChrgReq : Outport
  wires:
  Data Type Conversion/1 -> CAN2_LVSilentChrgReq/1
  LVSilentChrgReq/1 -> Data Type Conversion/1

== system halout/HAL_OUT/CAN2/FD2_CE100_0_0x117/LVSilentChrgSta ==
  LVSilentChrgSta : Inport
  Data Type Conversion : DataTypeConversion  OutDataTypeStr=uint8  RndMeth=Round
  CAN2_LVSilentChrgSta : Outport
  wires:
  Data Type Conversion/1 -> CAN2_LVSilentChrgSta/1
  LVSilentChrgSta/1 -> Data Type Conversion/1

== system halout/HAL_OUT/CAN2/FD2_CE100_0_0x117/LVSysErrPwrOutpErr ==
  LVSysErrPwrOutpErr : Inport
  Data Type Conversion : DataTypeConversion  OutDataTypeStr=uint8  RndMeth=Round
  CAN2_LVSysErr_PwrOutpErr : Outport
  wires:
  Data Type Conversion/1 -> CAN2_LVSysErr_PwrOutpErr/1
  LVSysErrPwrOutpErr/1 -> Data Type Conversion/1

== system halout/HAL_OUT/CAN2/FD2_CE100_0_0x117/LimphomeAct ==
  LimphomeAct : Inport
  Data Type Conversion : DataTypeConversion  OutDataTypeStr=uint8  RndMeth=Round
  CAN2_LimphomeAct : Outport
  wires:
  Data Type Conversion/1 -> CAN2_LimphomeAct/1
  LimphomeAct/1 -> Data Type Conversion/1

== system halout/HAL_OUT/CAN2/FD2_CE100_0_0x117/LockSetting ==
  LockSetting : Inport
  Data Type Conversion : DataTypeConversion  OutDataTypeStr=uint8  RndMeth=Round
  CAN2_LockSetting : Outport
  wires:
  Data Type Conversion/1 -> CAN2_LockSetting/1
  LockSetting/1 -> Data Type Conversion/1

== system halout/HAL_OUT/CAN2/FD2_CE100_0_0x117/MCUActDisFail ==
  MCUActDisFail : Inport
  Data Type Conversion : DataTypeConversion  OutDataTypeStr=uint8  RndMeth=Round
  CAN2_MCUActDisFail : Outport
  wires:
  Data Type Conversion/1 -> CAN2_MCUActDisFail/1
  MCUActDisFail/1 -> Data Type Conversion/1

== system halout/HAL_OUT/CAN2/FD2_CE100_0_0x117/MSACrlSta ==
  MSACrlSta : Inport
  Data Type Conversion : DataTypeConversion  OutDataTypeStr=uint8  RndMeth=Round
  CAN2_MSA_Crl_Sta : Outport
  wires:
  Data Type Conversion/1 -> CAN2_MSA_Crl_Sta/1
  MSACrlSta/1 -> Data Type Conversion/1

== system halout/HAL_OUT/CAN2/FD2_CE100_0_0x117/MeterIndSpeedraw32 ==
  MeterIndSpeedraw32 : Inport
  Data Type Conversion : DataTypeConversion  OutDataTypeStr=uint8  RndMeth=Round
  CAN2_MeterIndSpeed_raw32 : Outport
  wires:
  Data Type Conversion/1 -> CAN2_MeterIndSpeed_raw32/1
  MeterIndSpeedraw32/1 -> Data Type Conversion/1

== system halout/HAL_OUT/CAN2/FD2_CE100_0_0x117/PASStaFSys ==
  PASStaFSys : Inport
  Data Type Conversion : DataTypeConversion  OutDataTypeStr=uint8  RndMeth=Round
  CAN2_PAS_Sta_F_Sys : Outport
  wires:
  Data Type Conversion/1 -> CAN2_PAS_Sta_F_Sys/1
  PASStaFSys/1 -> Data Type Conversion/1

== system halout/HAL_OUT/CAN2/FD2_CE100_0_0x117/PosLamp ==
  PosLamp : Inport
  Data Type Conversion : DataTypeConversion  OutDataTypeStr=uint8  RndMeth=Round
  CAN2_PosLamp : Outport
  wires:
  Data Type Conversion/1 -> CAN2_PosLamp/1
  PosLamp/1 -> Data Type Conversion/1

== system halout/HAL_OUT/CAN2/FD2_CE100_0_0x117/PsDoorSW ==
  PsDoorSW : Inport
  Data Type Conversion : DataTypeConversion  OutDataTypeStr=uint8  RndMeth=Round
  CAN2_PsDoorSW : Outport
  wires:
  Data Type Conversion/1 -> CAN2_PsDoorSW/1
  PsDoorSW/1 -> Data Type Conversion/1

== system halout/HAL_OUT/CAN2/FD2_CE100_0_0x117/PwrSta ==
  PwrSta : Inport
  Data Type Conversion : DataTypeConversion  OutDataTypeStr=uint8  RndMeth=Round
  CAN2_PwrSta : Outport
  wires:
  Data Type Conversion/1 -> CAN2_PwrSta/1
  PwrSta/1 -> Data Type Conversion/1

== system halout/HAL_OUT/CAN2/FD2_CE100_0_0x117/PwrStaErr ==
  PwrStaErr : Inport
  Data Type Conversion : DataTypeConversion  OutDataTypeStr=uint8  RndMeth=Round
  CAN2_PwrStaErr : Outport
  wires:
  Data Type Conversion/1 -> CAN2_PwrStaErr/1
  PwrStaErr/1 -> Data Type Conversion/1

== system halout/HAL_OUT/CAN2/FD2_CE100_0_0x117/PwrStaONTOIVIPopReq ==
  PwrStaONTOIVIPopReq : Inport
  Data Type Conversion : DataTypeConversion  OutDataTypeStr=uint8  RndMeth=Round
  CAN2_PwrStaONTOIVIPopReq : Outport
  wires:
  Data Type Conversion/1 -> CAN2_PwrStaONTOIVIPopReq/1
  PwrStaONTOIVIPopReq/1 -> Data Type Conversion/1

== system halout/HAL_OUT/CAN2/FD2_CE100_0_0x117/PwrStaONTOIVIPopT ==
  PwrStaONTOIVIPopT : Inport
  Data Type Conversion : DataTypeConversion  OutDataTypeStr=uint16  RndMeth=Round
  CAN2_PwrStaONTOIVIPopT : Outport
  wires:
  Data Type Conversion/1 -> CAN2_PwrStaONTOIVIPopT/1
  PwrStaONTOIVIPopT/1 -> Data Type Conversion/1

== system halout/HAL_OUT/CAN2/FD2_CE100_0_0x117/RBSD ==
  RBSD : Inport
  Data Type Conversion : DataTypeConversion  OutDataTypeStr=uint8  RndMeth=Round
  CAN2_RBSD : Outport
  wires:
  Data Type Conversion/1 -> CAN2_RBSD/1
  RBSD/1 -> Data Type Conversion/1

== system halout/HAL_OUT/CAN2/FD2_CE100_0_0x117/RDRL ==
  RDRL : Inport
  Data Type Conversion : DataTypeConversion  OutDataTypeStr=uint8  RndMeth=Round
  CAN2_RDRL : Outport
  wires:
  Data Type Conversion/1 -> CAN2_RDRL/1
  RDRL/1 -> Data Type Conversion/1

== system halout/HAL_OUT/CAN2/FD2_CE100_0_0x117/RLDoorSW ==
  RLDoorSW : Inport
  Data Type Conversion : DataTypeConversion  OutDataTypeStr=uint8  RndMeth=Round
  CAN2_RLDoorSW : Outport
  wires:
  Data Type Conversion/1 -> CAN2_RLDoorSW/1
  RLDoorSW/1 -> Data Type Conversion/1

== system halout/HAL_OUT/CAN2/FD2_CE100_0_0x117/RRDoorSW ==
  RRDoorSW : Inport
  Data Type Conversion : DataTypeConversion  OutDataTypeStr=uint8  RndMeth=Round
  CAN2_RRDoorSW : Outport
  wires:
  Data Type Conversion/1 -> CAN2_RRDoorSW/1
  RRDoorSW/1 -> Data Type Conversion/1

== system halout/HAL_OUT/CAN2/FD2_CE100_0_0x117/RTurnLP ==
  RTurnLP : Inport
  Data Type Conversion : DataTypeConversion  OutDataTypeStr=uint8  RndMeth=Round
  CAN2_RTurnLP : Outport
  wires:
  Data Type Conversion/1 -> CAN2_RTurnLP/1
  RTurnLP/1 -> Data Type Conversion/1

== system halout/HAL_OUT/CAN2/FD2_CE100_0_0x117/ReqInternalV2LStatusLamp ==
  ReqInternalV2LStatusLamp : Inport
  Data Type Conversion : DataTypeConversion  OutDataTypeStr=uint8  RndMeth=Round
  CAN2_Req_Internal_V2L_Status_Lamp : Outport
  wires:
  Data Type Conversion/1 -> CAN2_Req_Internal_V2L_Status_Lamp/1
  ReqInternalV2LStatusLamp/1 -> Data Type Conversion/1

== system halout/HAL_OUT/CAN2/FD2_CE100_0_0x117/ReqV2LIVIPopup ==
  ReqV2LIVIPopup : Inport
  Data Type Conversion : DataTypeConversion  OutDataTypeStr=uint8  RndMeth=Round
  CAN2_Req_V2L_IVI_Popup : Outport
  wires:
  Data Type Conversion/1 -> CAN2_Req_V2L_IVI_Popup/1
  ReqV2LIVIPopup/1 -> Data Type Conversion/1

== system halout/HAL_OUT/CAN2/FD2_CE100_0_0x117/ReqV2LSwOn ==
  ReqV2LSwOn : Inport
  Data Type Conversion : DataTypeConversion  OutDataTypeStr=uint8  RndMeth=Round
  CAN2_Req_V2LSwOn : Outport
  wires:
  Data Type Conversion/1 -> CAN2_Req_V2LSwOn/1
  ReqV2LSwOn/1 -> Data Type Conversion/1

== system halout/HAL_OUT/CAN2/FD2_CE100_0_0x117/ReverseLamp ==
  ReverseLamp : Inport
  Data Type Conversion : DataTypeConversion  OutDataTypeStr=uint8  RndMeth=Round
  CAN2_ReverseLamp : Outport
  wires:
  Data Type Conversion/1 -> CAN2_ReverseLamp/1
  ReverseLamp/1 -> Data Type Conversion/1

== system halout/HAL_OUT/CAN2/FD2_CE100_0_0x117/RrDefog ==
  RrDefog : Inport
  Data Type Conversion : DataTypeConversion  OutDataTypeStr=uint8  RndMeth=Round
  CAN2_Rr_Defog : Outport
  wires:
  Data Type Conversion/1 -> CAN2_Rr_Defog/1
  RrDefog/1 -> Data Type Conversion/1

== system halout/HAL_OUT/CAN2/FD2_CE100_0_0x117/RrFogLamp ==
  RrFogLamp : Inport
  Data Type Conversion : DataTypeConversion  OutDataTypeStr=uint8  RndMeth=Round
  CAN2_Rr_FogLamp : Outport
  wires:
  Data Type Conversion/1 -> CAN2_Rr_FogLamp/1
  RrFogLamp/1 -> Data Type Conversion/1

== system halout/HAL_OUT/CAN2/FD2_CE100_0_0x117/ShiftGearPosn ==
  ShiftGearPosn : Inport
  Data Type Conversion : DataTypeConversion  OutDataTypeStr=uint8  RndMeth=Round
  CAN2_ShiftGearPosn : Outport
  wires:
  Data Type Conversion/1 -> CAN2_ShiftGearPosn/1
  ShiftGearPosn/1 -> Data Type Conversion/1

== system halout/HAL_OUT/CAN2/FD2_CE100_0_0x117/SysAllowReadySta ==
  SysAllowReadySta : Inport
  Data Type Conversion : DataTypeConversion  OutDataTypeStr=uint8  RndMeth=Round
  CAN2_SysAllowReadySta : Outport
  wires:
  Data Type Conversion/1 -> CAN2_SysAllowReadySta/1
  SysAllowReadySta/1 -> Data Type Conversion/1

== system halout/HAL_OUT/CAN2/FD2_CE100_0_0x117/SysPwrSta ==
  SysPwrSta : Inport
  Data Type Conversion : DataTypeConversion  OutDataTypeStr=uint8  RndMeth=Round
  CAN2_SysPwrSta : Outport
  wires:
  Data Type Conversion/1 -> CAN2_SysPwrSta/1
  SysPwrSta/1 -> Data Type Conversion/1

== system halout/HAL_OUT/CAN2/FD2_CE100_0_0x117/TailgateSW ==
  TailgateSW : Inport
  Data Type Conversion : DataTypeConversion  OutDataTypeStr=uint8  RndMeth=Round
  CAN2_Tailgate_SW : Outport
  wires:
  Data Type Conversion/1 -> CAN2_Tailgate_SW/1
  TailgateSW/1 -> Data Type Conversion/1

== system halout/HAL_OUT/CAN2/FD2_CE100_0_0x117/VCUBrkSWSta ==
  VCUBrkSWSta : Inport
  Data Type Conversion : DataTypeConversion  OutDataTypeStr=uint8  RndMeth=Round
  CAN2_VCUBrkSWSta : Outport
  wires:
  Data Type Conversion/1 -> CAN2_VCUBrkSWSta/1
  VCUBrkSWSta/1 -> Data Type Conversion/1

== system halout/HAL_OUT/CAN2/FD2_CE100_0_0x117/VCUFLDoorSta ==
  VCUFLDoorSta : Inport
  Data Type Conversion : DataTypeConversion  OutDataTypeStr=uint8  RndMeth=Round
  CAN2_VCUFLDoorSta : Outport
  wires:
  Data Type Conversion/1 -> CAN2_VCUFLDoorSta/1
  VCUFLDoorSta/1 -> Data Type Conversion/1

== system halout/HAL_OUT/CAN2/FD2_CE100_0_0x117/VCUFRDoorSta ==
  VCUFRDoorSta : Inport
  Data Type Conversion : DataTypeConversion  OutDataTypeStr=uint8  RndMeth=Round
  CAN2_VCUFRDoorSta : Outport
  wires:
  Data Type Conversion/1 -> CAN2_VCUFRDoorSta/1
  VCUFRDoorSta/1 -> Data Type Conversion/1

== system halout/HAL_OUT/CAN2/FD2_CE100_0_0x117/VCUHoodSWSta ==
  VCUHoodSWSta : Inport
  Data Type Conversion : DataTypeConversion  OutDataTypeStr=uint8  RndMeth=Round
  CAN2_VCUHoodSWSta : Outport
  wires:
  Data Type Conversion/1 -> CAN2_VCUHoodSWSta/1
  VCUHoodSWSta/1 -> Data Type Conversion/1

== system halout/HAL_OUT/CAN2/FD2_CE100_0_0x117/VCUOPDHold ==
  VCUOPDHold : Inport
  Data Type Conversion : DataTypeConversion  OutDataTypeStr=uint8  RndMeth=Round
  CAN2_VCU_OPDHold : Outport
  wires:
  Data Type Conversion/1 -> CAN2_VCU_OPDHold/1
  VCUOPDHold/1 -> Data Type Conversion/1

== system halout/HAL_OUT/CAN2/FD2_CE100_0_0x117/VCURLDoorSta ==
  VCURLDoorSta : Inport
  Data Type Conversion : DataTypeConversion  OutDataTypeStr=uint8  RndMeth=Round
  CAN2_VCURLDoorSta : Outport
  wires:
  Data Type Conversion/1 -> CAN2_VCURLDoorSta/1
  VCURLDoorSta/1 -> Data Type Conversion/1

== system halout/HAL_OUT/CAN2/FD2_CE100_0_0x117/VCURRDoorSta ==
  VCURRDoorSta : Inport
  Data Type Conversion : DataTypeConversion  OutDataTypeStr=uint8  RndMeth=Round
  CAN2_VCURRDoorSta : Outport
  wires:
  Data Type Conversion/1 -> CAN2_VCURRDoorSta/1
  VCURRDoorSta/1 -> Data Type Conversion/1

== system halout/HAL_OUT/CAN2/FD2_CE100_0_0x117/VCUTailgateSWSta ==
  VCUTailgateSWSta : Inport
  Data Type Conversion : DataTypeConversion  OutDataTypeStr=uint8  RndMeth=Round
  CAN2_VCUTailgateSWSta : Outport
  wires:
  Data Type Conversion/1 -> CAN2_VCUTailgateSWSta/1
  VCUTailgateSWSta/1 -> Data Type Conversion/1

== system halout/HAL_OUT/CAN2/FD2_CE100_0_0x117/VehMalfunLevel ==
  VehMalfunLevel : Inport
  Data Type Conversion : DataTypeConversion  OutDataTypeStr=uint8  RndMeth=Round
  CAN2_VehMalfunLevel : Outport
  wires:
  Data Type Conversion/1 -> CAN2_VehMalfunLevel/1
  VehMalfunLevel/1 -> Data Type Conversion/1

== system halout/HAL_OUT/CAN2/FD2_CE100_0_0x117/XWDMode ==
  XWDMode : Inport
  Data Type Conversion : DataTypeConversion  OutDataTypeStr=uint8  RndMeth=Round
  CAN2_XWDMode : Outport
  wires:
  Data Type Conversion/1 -> CAN2_XWDMode/1
  XWDMode/1 -> Data Type Conversion/1

== system halout/HAL_OUT/CAN2/FD2_CE100_0_0x117/sigAirIntenZon1St ==
  sigAirIntenZon1St : Inport
  Data Type Conversion : DataTypeConversion  OutDataTypeStr=uint8  RndMeth=Round
  CAN2_sigAirIntenZon1St : Outport
  wires:
  Data Type Conversion/1 -> CAN2_sigAirIntenZon1St/1
  sigAirIntenZon1St/1 -> Data Type Conversion/1

== system halout/HAL_OUT/CAN2/FD2_CE100_0_0x117/sigAirIntenZon3St ==
  sigAirIntenZon3St : Inport
  Data Type Conversion : DataTypeConversion  OutDataTypeStr=uint8  RndMeth=Round
  CAN2_sigAirIntenZon3St : Outport
  wires:
  Data Type Conversion/1 -> CAN2_sigAirIntenZon3St/1
  sigAirIntenZon3St/1 -> Data Type Conversion/1
